simulink model "arduino_matlab_codegen"  (R2025b)
settings: Solver=FixedStepDiscrete  StartTime=0.0  StopTime=10.0  RelTol=1e-3  EnableMultiTasking=on
settings Model: SimulationMode=external  ExtModeTrigDuration=2  Creator=The MathWorks, Inc.  LastModifiedBy=The MathWorks, Inc.
settings SolverCC: AlgebraicLoopSolver=TrustRegion
settings DataIOCC: ReturnWorkspaceOutputs=off
settings OptimizationCC: EnhancedBackFolding=on  PassReuseOutputArgsThreshold=0.0  MaxStackSize=64  OptimizeBlockOrder=speed  DifferentSizesBufferReuse=on  OptimizationCustomize=off
settings DebuggingCC: ParameterTunabilityLossMsg=error  UnconnectedInputMsg=warning  UnconnectedOutputMsg=warning  UnconnectedLineMsg=warning  SymbolicDimsDataTypeCodeGenerationDiagnostic=none
settings HardwareCC: ProdBitPerInt=16.0  ProdBitPerPointer=16.0  ProdBitPerSizeT=16.0  ProdBitPerPtrDiffT=16.0  ProdLargestAtomicFloat=None  ProdWordSize=8.0  ProdHWDeviceType=Atmel->AVR  UseEmbeddedCoderFeatures=off  UseSimulinkCoderFeatures=off
settings ModelReferenceCC: EnableRefExpFcnMdlSchedulingChecks=on
settings SFSimCC: MATLABDynamicMemAlloc=off
settings RTWCC: SystemTargetFile=ert.tlc  HardwareBoard=Arduino Mega 2560  TemplateMakefile=ert_default_tmf  GenerateReport=on  Toolchain=Arduino AVR  BuildConfiguration=Faster Runs  LaunchReport=on  GPUComputeCapability=3.5  Description=Embedded Coder
settings CodeAppCC: ForceParamTrailComments=on  OperatorAnnotations=on
settings ERTTargetCC: ExtModeStaticAllocSize=2048.0  InlinedParameterPlacement=Hierarchical  DynamicArrayContainerType=coder::array  ERTCustomFileBanners=off  SupportContinuousTime=on  SupportNonInlinedSFcns=on  RemoveResetFunc=off  SupportVariableSizeSignals=on  ModelStepFunctionPrototypeControlCompliant=off

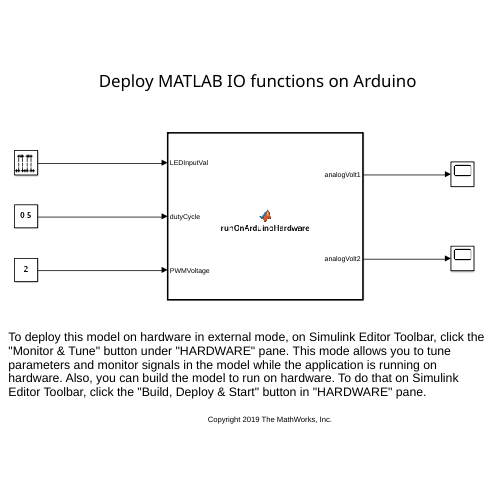
[thumbnail: Simulink's stored preview of the top-level diagram]
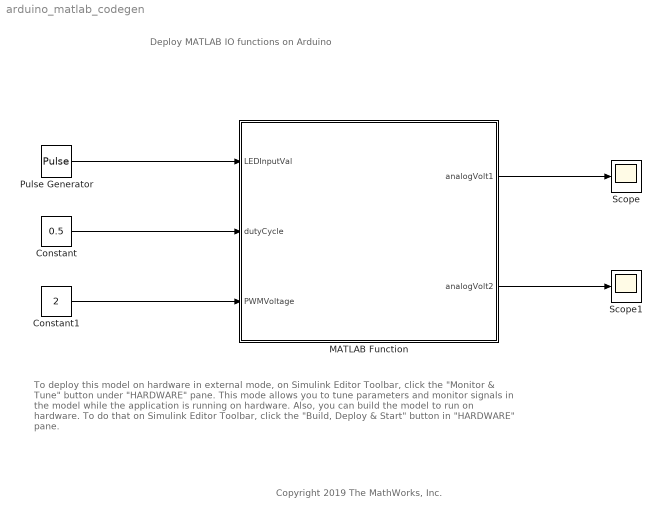
== system arduino_matlab_codegen ==
  note: To deploy this model on hardware in external mode, on Simulink Editor Toolbar, click the "Monitor & Tune" button under "HARDWARE" pane. This mode allows you to tune parameters and monitor signals in the model while the application is running on hardware. Also, you can build the model to run on hardware. To do that on Simulink Editor Toolbar, click the "Build, Deploy & Start" button in "HARDWARE" pane.
  note: Deploy MATLAB IO functions on Arduino
  note: Copyright 2019 The MathWorks, Inc.
  Constant : Constant  Value=0.5  SampleTime=-1
  Constant1 : Constant  Value=2  SampleTime=-1
  MATLAB Function : MATLAB Function  TreatAsAtomicUnit=on
  Pulse Generator : DiscretePulseGenerator  Period=10  PulseWidth=5  SampleTime=0.1
  Scope : Scope
      settings: ActiveDisplayYMinimum=-0.3794  ActiveDisplayYMaximum=5.56513
  Scope1 : Scope
      settings: ActiveDisplayYMinimum=-0.625  ActiveDisplayYMaximum=5.625
  wires:
  Pulse Generator/1 -> MATLAB Function/1(LEDInputVal)
  Constant/1 -> MATLAB Function/2(dutyCycle)
  Constant1/1 -> MATLAB Function/3(PWMVoltage)
  MATLAB Function/1(analogVolt1) -> Scope/1
  MATLAB Function/2(analogVolt2) -> Scope1/1

== matlab function arduino_matlab_codegen/MATLAB Function ==
  data: LEDInputVal input; analogVolt1 output; dutyCycle input; PWMVoltage input; analogVolt2 output
function [analogVolt1, analogVolt2] = runOnArduinoHardware(LEDInputVal, dutyCycle, PWMVoltage)

% This MATLAB Function block accesses multiple peripherals. It sets the
% state of a LED pin based on the value it receives as input. Also, it
% takes duty cycle and PWM voltage as inputs and generates a PWM signals
% accordingly. If those two PWM pins are connected to two analog pins (A1
% and A2 in this example), the PWM signal can be read by those analog pins.

%   Copyright 2019 The MathWorks, Inc.  

%% Initialize the variables
persistent arduinoObj;
ledPin = "D13";
pwmPin1 = "D3";
pwmPin2 = "D5";
analogPin1 = "A1";
analogPin2 = "A2";

%% create arduino object and configure the corresponding pins
if(isempty(arduinoObj))
    arduinoObj =  arduino();
    arduinoObj.configurePin(ledPin, 'DigitalOutput');
    arduinoObj.configurePin(analogPin1, 'AnalogInput');
    arduinoObj.configurePin(analogPin2, 'AnalogInput');
    arduinoObj.configurePin(pwmPin1, 'PWM');
    arduinoObj.configurePin(pwmPin2, 'PWM');
end

%% Access the peripherals
arduinoObj.writeDigitalPin(ledPin, LEDInputVal);
arduinoObj.writePWMDutyCycle(pwmPin1, dutyCycle);
arduinoObj.writePWMVoltage(pwmPin2, PWMVoltage);
analogVolt1 = arduinoObj.readVoltage(analogPin1);
analogVolt2 = arduinoObj.readVoltage(analogPin2);

%% [EOF]
